simulink model "SISTEMAP3"  (R2025b)
settings: Solver=ode23t  StartTime=0.0  StopTime=10.0  RelTol=1e-3
libraries: slpidlib x2
settings DataIOCC: ReturnWorkspaceOutputs=off  TimeSaveName=t
settings DebuggingCC: AlgebraicLoopMsg=none  ArtificialAlgebraicLoopMsg=none  MaxConsecutiveZCsMsg=none

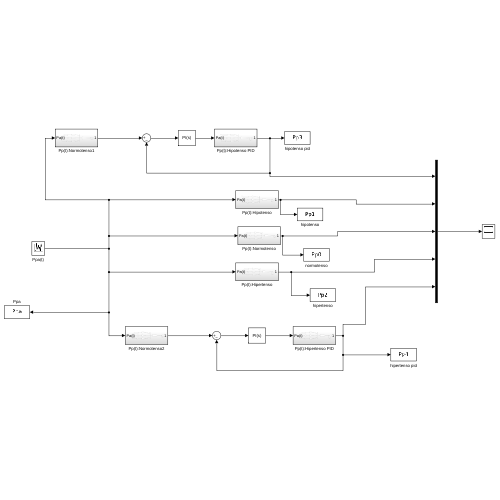
[thumbnail: Simulink's stored preview of the top-level diagram]
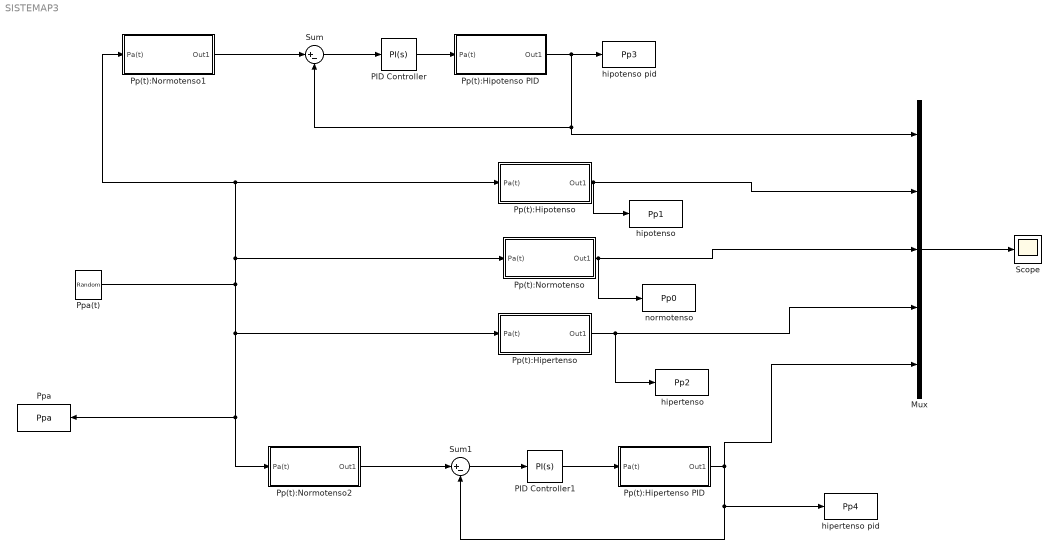
== system SISTEMAP3 ==
  Mux : Mux  Inputs=5
  PID Controller : slpidlib/PID Controller  Controller=PI  Form=Parallel  TimeDomain=Continuous-time  UseExternalTs=off  SampleTime=-1  IntegratorMethod=Forward Euler  FilterMethod=Forward Euler  ControllerParametersSource=internal  P=0.000103333333161111  I=41686938.2080771  UseKiTs=off  D=1  UseExternalDerivativeSource=off  N=1  UseFilter=on  TunerSelectOption=Transfer Function Based (PID Tuner App)  InitialConditionSource=internal  InitialConditionForIntegrator=0  InitialConditionForFilter=0  DifferentiatorICPrevScaledInput=0  ExternalReset=none  TrackingMode=off  Kt=1  LimitOutput=off  SatLimitsSource=internal  UpperSaturationLimit=inf  LowerSaturationLimit=-inf  LinearizeAsGain=on  AntiWindupMode=none  Kb=1  LimitIntegrator=off  UpperIntegratorSaturationLimit=inf  LowerIntegratorSaturationLimit=-inf  POutMin=[]  POutMax=[]  IOutMin=[]  IOutMax=[]  DOutMin=[]  DOutMax=[]  NOutMin=[]  NOutMax=[]  SumOutMin=[]  SumOutMax=[]  SaturationOutMin=[]  SaturationOutMax=[]  PParamMin=[]  PParamMax=[]  IParamMin=[]  IParamMax=[]  DParamMin=[]  DParamMax=[]  NParamMin=[]  NParamMax=[]  KbParamMin=[]  KbParamMax=[]  KtParamMin=[]  KtParamMax=[]  KbOutMin=[]  KbOutMax=[]  KtOutMin=[]  KtOutMax=[]  IntegratorOutMin=[]  IntegratorOutMax=[]  FilterOutMin=[]  FilterOutMax=[]  SumI1OutMin=[]  SumI1OutMax=[]  SumI2OutMin=[]  SumI2OutMax=[]  SumI3OutMin=[]  SumI3OutMax=[]  SumI4OutMin=[]  SumI4OutMax=[]  SumDOutMin=[]  SumDOutMax=[]  DifferentiatorOutMin=[]  DifferentiatorOutMax=[]  FilterDiffOutCoefMin=[]  FilterDiffOutCoefMax=[]  ReciprocalOutMin=[]  ReciprocalOutMax=[]  SumDenOutMin=[]  SumDenOutMax=[]  SumNumOutMin=[]  SumNumOutMax=[]  DivideOutMin=[]  DivideOutMax=[]  UdiffTsProdOutMin=[]  UdiffTsProdOutMax=[]  NTsProdOutMin=[]  NTsProdOutMax=[]  UintegralTsProdOutMin=[]  UintegralTsProdOutMax=[]  UngainTsProdOutMin=[]  UngainTsProdOutMax=[]  ClampingZeroOutDataTypeStr=Inherit: Inherit via back propagation  ClampingZeroOutMin=[]  ClampingZeroOutMax=[]  FilterDenConstantOutDataTypeStr=Inherit: Inherit via back propagation  FilterDenConstantOutMin=[]  FilterDenConstantOutMax=[]  PCopyOutDataTypeStr=Inherit: Inherit via back propagation  PCopyOutMin=[]  PCopyOutMax=[]  NCopyOutDataTypeStr=Inherit: Inherit via back propagation  NCopyOutMin=[]  NCopyOutMax=[]  IntegratorContinuousStateAttributes=''  IntegratorStateMustResolveToSignalObject=off  IntegratorRTWStateStorageClass=Auto  FilterContinuousStateAttributes=''  FilterStateMustResolveToSignalObject=off  FilterRTWStateStorageClass=Auto  ParallelPVariant=InternalParameters  IdealPVariant=Disabled  IVariant=InternalParameters  DVariant=Disabled  IntegratorVariant=Continuous  SatVariant=Disabled  AWVariant=Passthrough  PCopyVariant=Disabled  TRVariant=Disabled  FdbkBlocksVariant=Forward  IdealPFdbkVariant=Disabled  SatFdbkVariant=Disabled  DerivativeFilterVariant=Disabled  NVariant=Disabled  NCopyVariant=Disabled_SignalSpec  FilterICVariant=Disabled  IntegratorICVariant=InternalICs  ExternalResetVariant=Disabled  TRSumVariant=Passthrough  SumFdbkVariant=Disabled  SumVariant=Sum_PI  TsampFilterVariant=InternalTs  TsampNgainVariant=Passthrough  TsampIntegralVariant=Disabled_SignalSpec  ExternalSaturationOutDataTypeStr=Inherit: Same as second input  DerivativeSourceVariant=Disabled  PreIntVariant=InternalPreInt
  PID Controller1 : slpidlib/PID Controller  Controller=PI  Form=Parallel  TimeDomain=Continuous-time  UseExternalTs=off  SampleTime=-1  IntegratorMethod=Forward Euler  FilterMethod=Forward Euler  ControllerParametersSource=internal  P=10  I=4132.36404565657  UseKiTs=off  D=1  UseExternalDerivativeSource=off  N=1  UseFilter=on  TunerSelectOption=Transfer Function Based (PID Tuner App)  InitialConditionSource=internal  InitialConditionForIntegrator=0  InitialConditionForFilter=0  DifferentiatorICPrevScaledInput=0  ExternalReset=none  TrackingMode=off  Kt=1  LimitOutput=off  SatLimitsSource=internal  UpperSaturationLimit=inf  LowerSaturationLimit=-inf  LinearizeAsGain=on  AntiWindupMode=none  Kb=1  LimitIntegrator=off  UpperIntegratorSaturationLimit=inf  LowerIntegratorSaturationLimit=-inf  POutMin=[]  POutMax=[]  IOutMin=[]  IOutMax=[]  DOutMin=[]  DOutMax=[]  NOutMin=[]  NOutMax=[]  SumOutMin=[]  SumOutMax=[]  SaturationOutMin=[]  SaturationOutMax=[]  PParamMin=[]  PParamMax=[]  IParamMin=[]  IParamMax=[]  DParamMin=[]  DParamMax=[]  NParamMin=[]  NParamMax=[]  KbParamMin=[]  KbParamMax=[]  KtParamMin=[]  KtParamMax=[]  KbOutMin=[]  KbOutMax=[]  KtOutMin=[]  KtOutMax=[]  IntegratorOutMin=[]  IntegratorOutMax=[]  FilterOutMin=[]  FilterOutMax=[]  SumI1OutMin=[]  SumI1OutMax=[]  SumI2OutMin=[]  SumI2OutMax=[]  SumI3OutMin=[]  SumI3OutMax=[]  SumI4OutMin=[]  SumI4OutMax=[]  SumDOutMin=[]  SumDOutMax=[]  DifferentiatorOutMin=[]  DifferentiatorOutMax=[]  FilterDiffOutCoefMin=[]  FilterDiffOutCoefMax=[]  ReciprocalOutMin=[]  ReciprocalOutMax=[]  SumDenOutMin=[]  SumDenOutMax=[]  SumNumOutMin=[]  SumNumOutMax=[]  DivideOutMin=[]  DivideOutMax=[]  UdiffTsProdOutMin=[]  UdiffTsProdOutMax=[]  NTsProdOutMin=[]  NTsProdOutMax=[]  UintegralTsProdOutMin=[]  UintegralTsProdOutMax=[]  UngainTsProdOutMin=[]  UngainTsProdOutMax=[]  ClampingZeroOutDataTypeStr=Inherit: Inherit via back propagation  ClampingZeroOutMin=[]  ClampingZeroOutMax=[]  FilterDenConstantOutDataTypeStr=Inherit: Inherit via back propagation  FilterDenConstantOutMin=[]  FilterDenConstantOutMax=[]  PCopyOutDataTypeStr=Inherit: Inherit via back propagation  PCopyOutMin=[]  PCopyOutMax=[]  NCopyOutDataTypeStr=Inherit: Inherit via back propagation  NCopyOutMin=[]  NCopyOutMax=[]  IntegratorContinuousStateAttributes=''  IntegratorStateMustResolveToSignalObject=off  IntegratorRTWStateStorageClass=Auto  FilterContinuousStateAttributes=''  FilterStateMustResolveToSignalObject=off  FilterRTWStateStorageClass=Auto  ParallelPVariant=InternalParameters  IdealPVariant=Disabled  IVariant=InternalParameters  DVariant=Disabled  IntegratorVariant=Continuous  SatVariant=Disabled  AWVariant=Passthrough  PCopyVariant=Disabled  TRVariant=Disabled  FdbkBlocksVariant=Forward  IdealPFdbkVariant=Disabled  SatFdbkVariant=Disabled  DerivativeFilterVariant=Disabled  NVariant=Disabled  NCopyVariant=Disabled_SignalSpec  FilterICVariant=Disabled  IntegratorICVariant=InternalICs  ExternalResetVariant=Disabled  TRSumVariant=Passthrough  SumFdbkVariant=Disabled  SumVariant=Sum_PI  TsampFilterVariant=InternalTs  TsampNgainVariant=Passthrough  TsampIntegralVariant=Disabled_SignalSpec  ExternalSaturationOutDataTypeStr=Inherit: Same as second input  DerivativeSourceVariant=Disabled  PreIntVariant=InternalPreInt
  Pp(t):Hipertenso : Subsystem
  Pp(t):Hipertenso PID : Subsystem
  Pp(t):Hipotenso : Subsystem
  Pp(t):Hipotenso PID : Subsystem
  Pp(t):Normotenso : Subsystem
  Pp(t):Normotenso1 : Subsystem
  Pp(t):Normotenso2 : Subsystem
  Ppa : ToWorkspace  VariableName=Ppa  SampleTime=-1
  Ppa(t) : UniformRandomNumber  Minimum=-0.2  Seed=106  SampleTime=0.5
  Scope : Scope
      settings: ActiveDisplayYMinimum=-0.32314698688612775  ActiveDisplayYMaximum=1.1154871758165368
  Sum : Sum  Inputs=|+-
  Sum1 : Sum  Inputs=|+-
  hipertenso : ToWorkspace  VariableName=Pp2  SampleTime=-1
  hipertenso pid : ToWorkspace  VariableName=Pp4  SampleTime=-1
  hipotenso : ToWorkspace  VariableName=Pp1  SampleTime=-1
  hipotenso pid : ToWorkspace  VariableName=Pp3  SampleTime=-1
  normotenso : ToWorkspace  VariableName=Pp0  SampleTime=-1
  wires:
  Mux/1 -> Scope/1
  Pp(t):Hipotenso PID/1(Out1) -> hipotenso pid/1, Sum/2, Mux/1
  Pp(t):Normotenso1/1(Out1) -> Sum/1
  Sum/1 -> PID Controller/1
  PID Controller/1 -> Pp(t):Hipotenso PID/1(Pa(t))
  Pp(t):Hipertenso/1(Out1) -> hipertenso/1, Mux/4
  Pp(t):Normotenso/1(Out1) -> normotenso/1, Mux/3
  Pp(t):Hipotenso/1(Out1) -> hipotenso/1, Mux/2
  Ppa(t)/1 -> Pp(t):Normotenso1/1(Pa(t)), Pp(t):Hipotenso/1(Pa(t)), Pp(t):Normotenso/1(Pa(t)), Ppa/1, Pp(t):Normotenso2/1(Pa(t)), Pp(t):Hipertenso/1(Pa(t))
  Sum1/1 -> PID Controller1/1
  Pp(t):Normotenso2/1(Out1) -> Sum1/1
  PID Controller1/1 -> Pp(t):Hipertenso PID/1(Pa(t))
  Pp(t):Hipertenso PID/1(Out1) -> Mux/5, hipertenso pid/1, Sum1/2

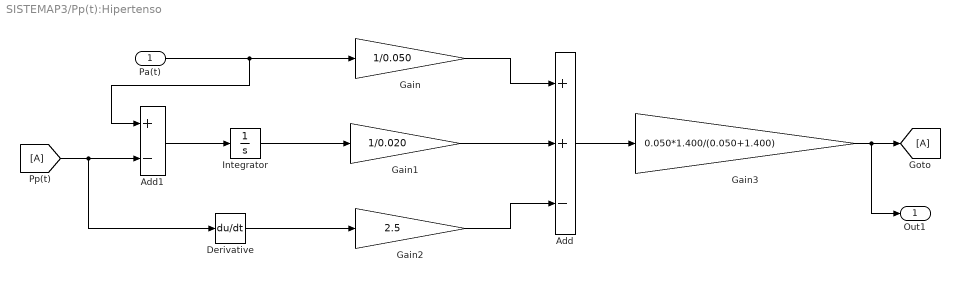
== system SISTEMAP3/Pp(t):Hipertenso ==
  Pa(t) : Inport
  Add : Sum  Inputs=++-
  Add1 : Sum  Inputs=+-
  Derivative : Derivative
  Gain : Gain  Gain=1/0.050
  Gain1 : Gain  Gain=1/0.020
  Gain2 : Gain  Gain=2.5
  Gain3 : Gain  Gain=0.050*1.400/(0.050+1.400)
  Goto : Goto
  Integrator : Integrator
  Pp(t) : From
  Out1 : Outport
  wires:
  Gain/1 -> Add/1
  Gain1/1 -> Add/2
  Gain2/1 -> Add/3
  Integrator/1 -> Gain1/1
  Derivative/1 -> Gain2/1
  Add1/1 -> Integrator/1
  Add/1 -> Gain3/1
  Pa(t)/1 -> Add1/1, Gain/1
  Pp(t)/1 -> Derivative/1, Add1/2
  Gain3/1 -> Out1/1, Goto/1

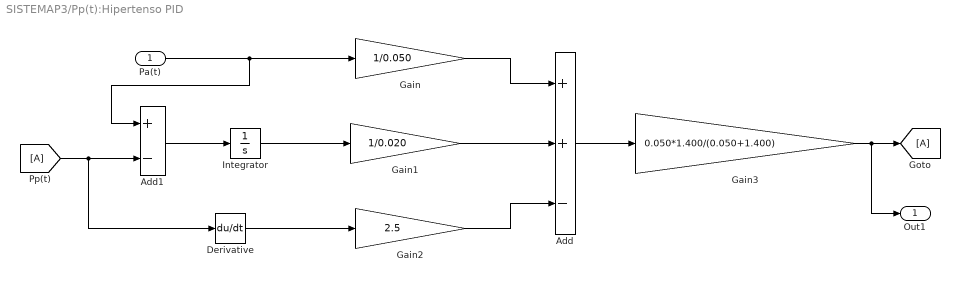
== system SISTEMAP3/Pp(t):Hipertenso PID ==
  Pa(t) : Inport
  Add : Sum  Inputs=++-
  Add1 : Sum  Inputs=+-
  Derivative : Derivative
  Gain : Gain  Gain=1/0.050
  Gain1 : Gain  Gain=1/0.020
  Gain2 : Gain  Gain=2.5
  Gain3 : Gain  Gain=0.050*1.400/(0.050+1.400)
  Goto : Goto
  Integrator : Integrator
  Pp(t) : From
  Out1 : Outport
  wires:
  Gain/1 -> Add/1
  Gain1/1 -> Add/2
  Gain2/1 -> Add/3
  Integrator/1 -> Gain1/1
  Derivative/1 -> Gain2/1
  Add1/1 -> Integrator/1
  Add/1 -> Gain3/1
  Pa(t)/1 -> Add1/1, Gain/1
  Pp(t)/1 -> Derivative/1, Add1/2
  Gain3/1 -> Out1/1, Goto/1

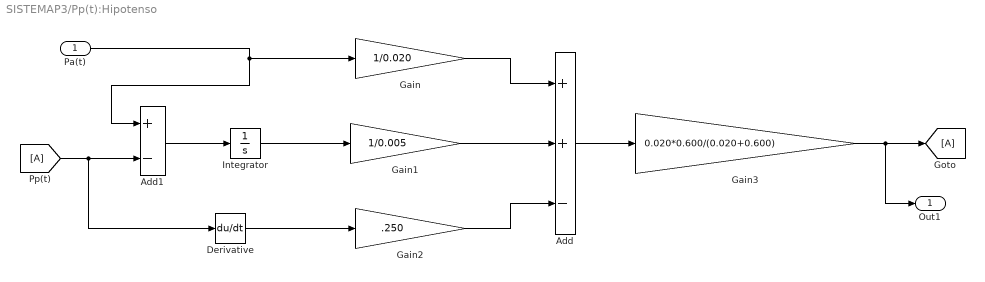
== system SISTEMAP3/Pp(t):Hipotenso ==
  Pa(t) : Inport
  Add : Sum  Inputs=++-
  Add1 : Sum  Inputs=+-
  Derivative : Derivative
  Gain : Gain  Gain=1/0.020
  Gain1 : Gain  Gain=1/0.005
  Gain2 : Gain  Gain=.250
  Gain3 : Gain  Gain=0.020*0.600/(0.020+0.600)
  Goto : Goto
  Integrator : Integrator
  Pp(t) : From
  Out1 : Outport
  wires:
  Gain/1 -> Add/1
  Gain1/1 -> Add/2
  Gain2/1 -> Add/3
  Integrator/1 -> Gain1/1
  Derivative/1 -> Gain2/1
  Add1/1 -> Integrator/1
  Add/1 -> Gain3/1
  Pa(t)/1 -> Add1/1, Gain/1
  Pp(t)/1 -> Derivative/1, Add1/2
  Gain3/1 -> Goto/1, Out1/1

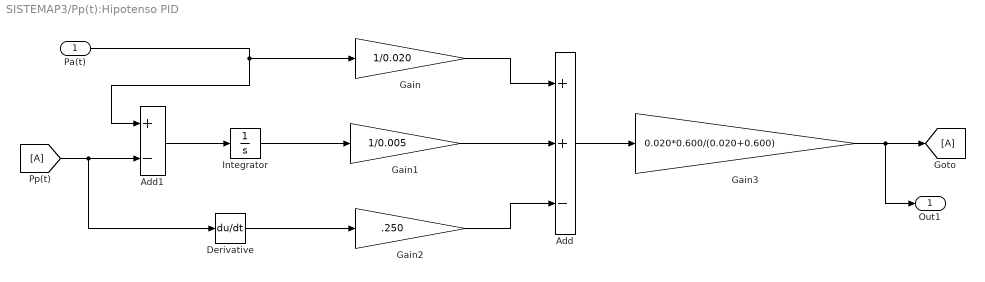
== system SISTEMAP3/Pp(t):Hipotenso PID ==
  Pa(t) : Inport
  Add : Sum  Inputs=++-
  Add1 : Sum  Inputs=+-
  Derivative : Derivative
  Gain : Gain  Gain=1/0.020
  Gain1 : Gain  Gain=1/0.005
  Gain2 : Gain  Gain=.250
  Gain3 : Gain  Gain=0.020*0.600/(0.020+0.600)
  Goto : Goto
  Integrator : Integrator
  Pp(t) : From
  Out1 : Outport
  wires:
  Gain/1 -> Add/1
  Gain1/1 -> Add/2
  Gain2/1 -> Add/3
  Integrator/1 -> Gain1/1
  Derivative/1 -> Gain2/1
  Add1/1 -> Integrator/1
  Add/1 -> Gain3/1
  Pa(t)/1 -> Add1/1, Gain/1
  Pp(t)/1 -> Derivative/1, Add1/2
  Gain3/1 -> Goto/1, Out1/1

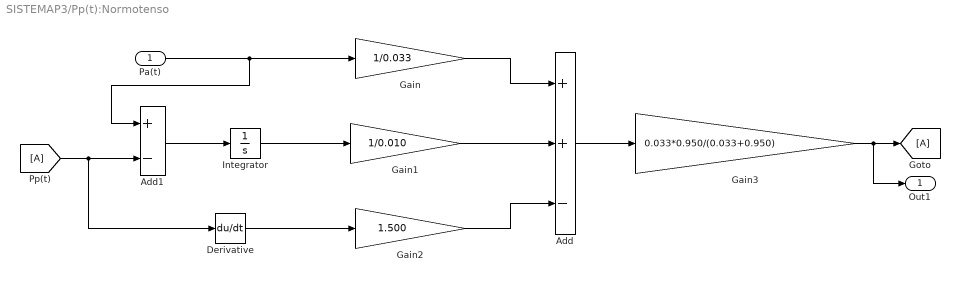
== system SISTEMAP3/Pp(t):Normotenso ==
  Pa(t) : Inport
  Add : Sum  Inputs=++-
  Add1 : Sum  Inputs=+-
  Derivative : Derivative
  Gain : Gain  Gain=1/0.033
  Gain1 : Gain  Gain=1/0.010
  Gain2 : Gain  Gain=1.500
  Gain3 : Gain  Gain=0.033*0.950/(0.033+0.950)
  Goto : Goto
  Integrator : Integrator
  Pp(t) : From
  Out1 : Outport
  wires:
  Gain/1 -> Add/1
  Gain1/1 -> Add/2
  Gain2/1 -> Add/3
  Integrator/1 -> Gain1/1
  Derivative/1 -> Gain2/1
  Add1/1 -> Integrator/1
  Add/1 -> Gain3/1
  Pa(t)/1 -> Add1/1, Gain/1
  Pp(t)/1 -> Derivative/1, Add1/2
  Gain3/1 -> Out1/1, Goto/1

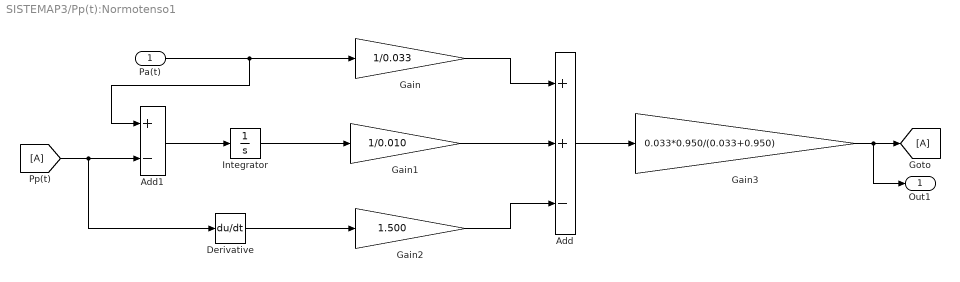
== system SISTEMAP3/Pp(t):Normotenso1 ==
  Pa(t) : Inport
  Add : Sum  Inputs=++-
  Add1 : Sum  Inputs=+-
  Derivative : Derivative
  Gain : Gain  Gain=1/0.033
  Gain1 : Gain  Gain=1/0.010
  Gain2 : Gain  Gain=1.500
  Gain3 : Gain  Gain=0.033*0.950/(0.033+0.950)
  Goto : Goto
  Integrator : Integrator
  Pp(t) : From
  Out1 : Outport
  wires:
  Gain/1 -> Add/1
  Gain1/1 -> Add/2
  Gain2/1 -> Add/3
  Integrator/1 -> Gain1/1
  Derivative/1 -> Gain2/1
  Add1/1 -> Integrator/1
  Add/1 -> Gain3/1
  Pa(t)/1 -> Add1/1, Gain/1
  Pp(t)/1 -> Derivative/1, Add1/2
  Gain3/1 -> Out1/1, Goto/1

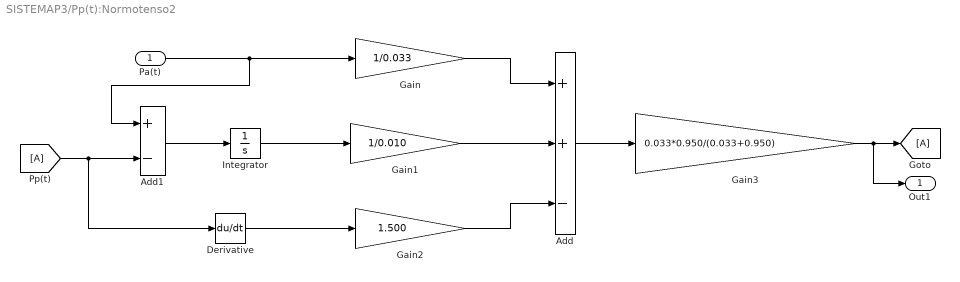
== system SISTEMAP3/Pp(t):Normotenso2 ==
  Pa(t) : Inport
  Add : Sum  Inputs=++-
  Add1 : Sum  Inputs=+-
  Derivative : Derivative
  Gain : Gain  Gain=1/0.033
  Gain1 : Gain  Gain=1/0.010
  Gain2 : Gain  Gain=1.500
  Gain3 : Gain  Gain=0.033*0.950/(0.033+0.950)
  Goto : Goto
  Integrator : Integrator
  Pp(t) : From
  Out1 : Outport
  wires:
  Gain/1 -> Add/1
  Gain1/1 -> Add/2
  Gain2/1 -> Add/3
  Integrator/1 -> Gain1/1
  Derivative/1 -> Gain2/1
  Add1/1 -> Integrator/1
  Add/1 -> Gain3/1
  Pa(t)/1 -> Add1/1, Gain/1
  Pp(t)/1 -> Derivative/1, Add1/2
  Gain3/1 -> Out1/1, Goto/1
